simulink model "SF012A_HysCmp"  (R2013b)
settings: Solver=FixedStepDiscrete  StartTime=0.0  StopTime=1  FixedStep=.002  RelTol=1e-3
values from neighbouring files (symbols this model uses):
  ARCHGLBPRM_2MILLISEC_SEC_F32 = DataDict.Constant    [SF012A_HysCmp_DataDict.m]
  EPSILON_ULS_F32 = DataDict.Constant    [SF012A_HysCmp_DataDict.m]
  FLTINJ_HYSCMP_HYSCMPCMD = DataDict.Constant    [SF012A_HysCmp_DataDict.m]
  HysCmpAssiInpLim = DataDict.Calibration    [SF012A_HysCmp_DataDict.m]
  HysCmpOutpLim = DataDict.Calibration    [SF012A_HysCmp_DataDict.m]
  HysCmpRevGain = DataDict.Calibration    [SF012A_HysCmp_DataDict.m]
  HysCmpRiseX = DataDict.Calibration    [SF012A_HysCmp_DataDict.m]
  HysCmpRiseY = DataDict.Calibration    [SF012A_HysCmp_DataDict.m]
  HYSRISEYLIM_ULS_F32 = DataDict.Constant    [SF012A_HysCmp_DataDict.m]
  HYSSATNLOWLIM_HWNWTMTR_F32 = DataDict.Constant    [SF012A_HysCmp_DataDict.m]
  SysGlbPrmSysTqRat = DataDict.ImprtdCal    [SF012A_HysCmp_DataDict.m]
libraries: FixdToFloat x18, FloatToFixd x14, LnrIntrpn x12, NxtrAbslt x10, NxtrLim x8, Fil x6, NxtrSign x5, simulink x2, NxtrMath x1, BilnrIntrpnMplX x1, NxtrMax x1
(part 1 of 2)
settings Model: Creator=TZ5743  LastModifiedBy=TZ5743
settings DataIOCC: LimitDataPoints=off  SaveFormat=Structure  ReturnWorkspaceOutputs=on
settings OptimizationCC: BlockReduction=off  InlineParams=on  ZeroExternalMemoryAtStartup=off  ZeroInternalMemoryAtStartup=off  OptimizeModelRefInitCode=on  LifeSpan=1
settings DebuggingCC: SignalInfNanChecking=error  SignalRangeChecking=warning  UnderspecifiedInitializationDetection=Simplified  SolverPrmCheckMsg=error  InheritedTsInSrcMsg=error  DiscreteInheritContinuousMsg=error  SingleTaskRateTransMsg=error  TasksWithSamePriorityMsg=error  SigSpecEnsureSampleTimeMsg=error  CheckMatrixSingularityMsg=error  IntegerOverflowMsg=error  ParameterUnderflowMsg=error  ParameterPrecisionLossMsg=error  ParameterTunabilityLossMsg=error  FixptConstUnderflowMsg=warning  FixptConstOverflowMsg=warning  VectorMatrixConversionMsg=error  SignalLabelMismatchMsg=error  UnconnectedInputMsg=error  UnconnectedOutputMsg=error  UnconnectedLineMsg=error  SFcnCompatibilityMsg=error  UniqueDataStoreMsg=warning  BusObjectLabelMismatch=error  RootOutportRequireBusObject=error  AssertControl=DisableAll  ModelReferenceIOMsg=error  ModelReferenceVersionMismatchMessage=warning  ModelReferenceIOMismatchMessage=error  ModelReferenceCSMismatchMessage=warning  ModelReferenceDataLoggingMessage=error  StateNameClashWarn=warning  StrictBusMsg=ErrorOnBusTreatedAsVector  NonBusSignalsTreatedAsBus=error  SFUnexpectedBacktrackingDiag=error  SFInvalidInputDataAccessInChartInitDiag=error  SFNoUnconditionalDefaultTransitionDiag=error  SFTransitionOutsideNaturalParentDiag=error  SFUnconditionalTransitionShadowingDiag=error  SFUndirectedBroadcastEventsDiag=error
settings ModelReferenceCC: ModelReferenceNumInstancesAllowed=Single
settings RTWCC: SystemTargetFile=autosar.tlc  GenCodeOnly=on  TemplateMakefile=ert_default_tmf  Description=AUTOSAR  GenerateReport=on  ProcessScript=autosar_make_rtw_hook  LaunchReport=on
settings CodeAppCC: GenerateComments=off  IgnoreCustomStorageClasses=off  CustomSymbolStrType=$N$R$M  CustomSymbolStrBlkIO=$N$M  SimulinkBlockComments=off
settings STFCustomTargetCC: ParMdlRefBuildCompliant=on  CompOptLevelCompliant=on  IncludeMdlTerminateFcn=off  CombineOutputUpdateFcns=on  SuppressErrorStatus=on  ERTFirstTimeCompliant=on  ERTCustomFileBanners=on  SupportNonFinite=off  SupportComplex=off  SupportContinuousTime=off  SupportNonInlinedSFcns=off  MATLABClassNameForMDSCustomization=Simulink.SoftwareTarget.ERTCustomization  AutosarCompliant=on  GRTInterface=off  SystemTargetFile=autosar.tlc
settings ERTTargetCC: CodeReplacementLibrary=ANSI_C  ConcurrentExecutionCompliant=off  IncludeMdlTerminateFcn=off  SuppressErrorStatus=on  SupportNonFinite=off  SupportComplex=off  ModelStepFunctionPrototypeControlCompliant=off  CPPClassGenCompliant=off  AutosarCompliant=on  InlinedParameterPlacement=NonHierarchical  ERTCustomFileTemplate=example_file_process.tlc  EnableUserReplacementTypes=on

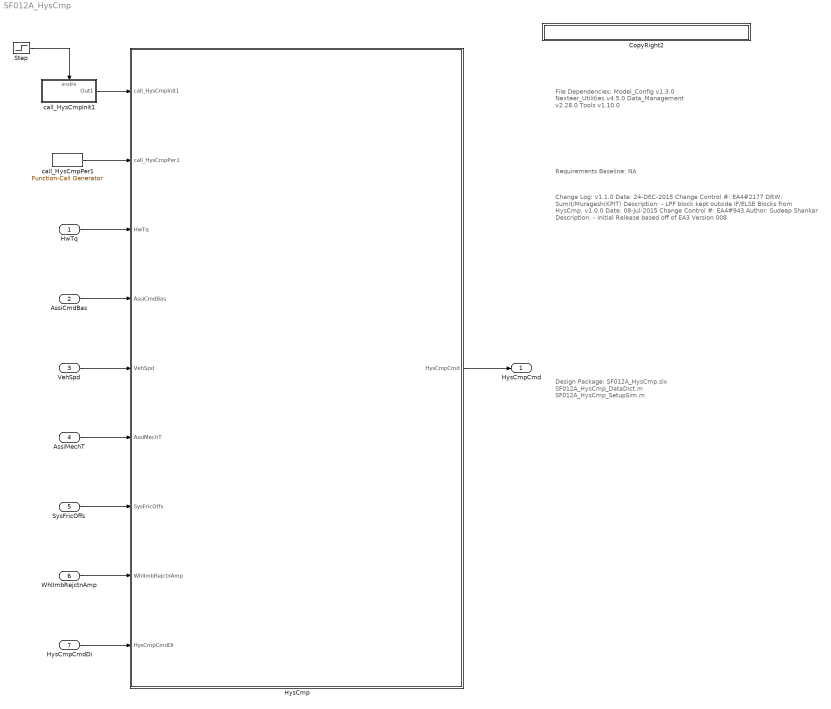
== system SF012A_HysCmp ==
  note: File Dependencies:
      |
      | Model_Config v1.3.0
      | Nexteer_Utilities v4.5.0
      | Data_Management v2.28.0
      | Tools v1.10.0
  note: Requirements Baseline: NA
  note: Change Log:
      | v1.1.0
      | Date: 24-DEC-2015
      | Change Control #: EA4#2177
      | DRW:  Sumit/Muragesh(KPIT)
      | Description:
      | -  LPF block kept outside IF/ELSE Blocks from HysCmp.
      |
      | v1.0.0
      | Date: 08-Jul-2015
      | Change Control #: EA4#943
      | Author:  Sudeep Shankar
      | Description:
      | - Initial Release based off of EA3 Version 008
  note: Design Package:
      |
      | SF012A_HysCmp.slx
      | SF012A_HysCmp_DataDict.m
      | SF012A_HysCmp_SetupSim.m
  HwTq : Inport
  AssiCmdBas : Inport  Port=2
  VehSpd : Inport  Port=3
  AssiMechT : Inport  Port=4
  SysFricOffs : Inport  Port=5
  WhlImbRejctnAmp : Inport  Port=6
  HysCmpCmdDi : Inport  Port=7
  CopyRight2 : Subsystem  Description=|  mask(Copyright Information){none=on}
      | Copyright info block.                                               
      |                                                                     
      | Place copyright information at the top of every subsystem in design.
      mask prompts: none "No parameters"
      mask help: Place copyright information at the top of every subsystem in design.
      mask Display:
      | NxtrConf = 'Nexteer Confidential';
      | 
      | sys = bdroot; %handle for the current model ("system")
      | first = get_param(sys,'Created');
      | if(isempty(first))
      |     first = datestr(now,'yyyy');
      | else
      |     first = first(end-3:end);  %year is last four digits
      | end
      | 
      | last = get_param(sys,'LastModifiedDate');
      | if isempty(last)
      |     last = datestr(now,'yyyy');
      | else
      |     last = last(end-3:end);
      | end
      | 
      | if strcmp(first,last)
      |     fprintf('%s -- Copyright %s Nexteer',NxtrConf,first)
      | else
      |     fprintf('%s -- %s%s- %s Nexteer',NxtrConf,char(169),first,last)
      | end
  HysCmp : Subsystem
  Step : Step  Time=.001  Before=1  After=0  SampleTime=0
  call_HysCmpInit1 : Subsystem  TreatAsAtomicUnit=on
  call_HysCmpPer1 : simulink/Ports & Subsystems/Function-Call Generator  RequirementInfo={} %GIDa_211e4458_5e3d_455a_8408_cf5f2d6f0325  sample_time=0.002  numberOfIterations=1
  HysCmpCmd : Outport
  wires:
  HwTq/1 -> HysCmp/3(HwTq)
  AssiCmdBas/1 -> HysCmp/4(AssiCmdBas)
  VehSpd/1 -> HysCmp/5(VehSpd)
  AssiMechT/1 -> HysCmp/6(AssiMechT)
  SysFricOffs/1 -> HysCmp/7(SysFricOffs)
  WhlImbRejctnAmp/1 -> HysCmp/8(WhlImbRejctnAmp)
  HysCmpCmdDi/1 -> HysCmp/9(HysCmpCmdDi)
  HysCmp/1(HysCmpCmd) -> HysCmpCmd/1
  call_HysCmpPer1/1 -> HysCmp/2(call_HysCmpPer1)
  call_HysCmpInit1/1(Out1) -> HysCmp/1(call_HysCmpInit1)
  Step/1 -> call_HysCmpInit1/Enable

== system SF012A_HysCmp/CopyRight2 ==

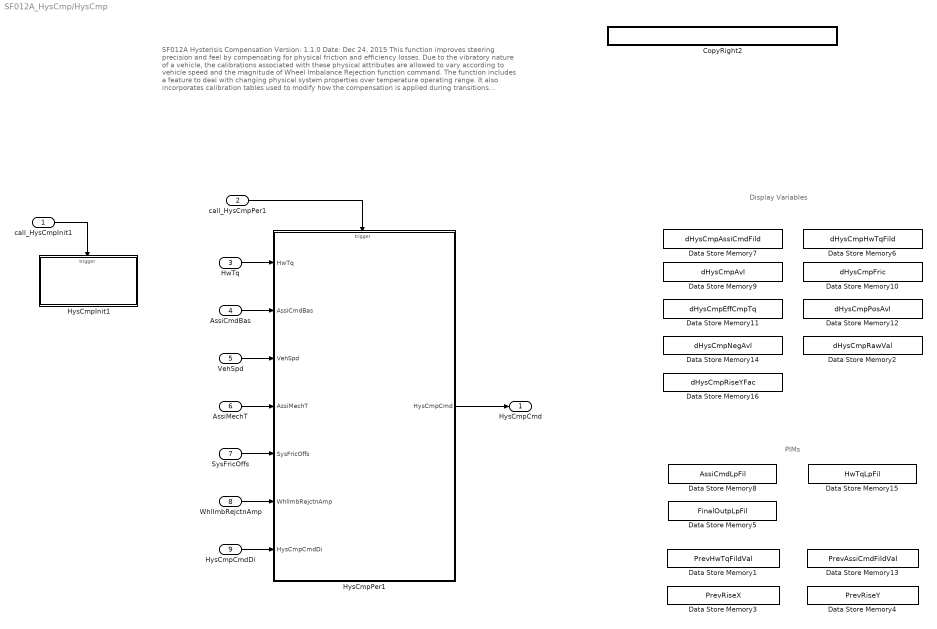
== system SF012A_HysCmp/HysCmp ==
  note: SF012A Hysterisis Compensation       Version: 1.1.0                                                        Date:  Dec 24, 2015
      |
      | This function improves steering precision and feel by compensating for physical friction and efficiency losses.
      | Due to the vibratory nature of a vehicle, the calibrations associated with these physical attributes are allowed
      | to vary according to vehicle speed and the magnitude of Wheel Imbalance Rejection function command. The function
      | includes a feature to deal with changing physical system properties over temperature operating range. It also
      | incorporates calibration tables used to modify how the compensation is applied during transitions between operating
      | quadrants and during periods of near-zero handwheel torque. Finally the function may be disabled for purposes of
      | bench testing
  note: PIMs
  note: Display Variables
  call_HysCmpInit1 : Inport
  call_HysCmpPer1 : Inport  Port=2
  HwTq : Inport  Port=3
  AssiCmdBas : Inport  Port=4
  VehSpd : Inport  Port=5
  AssiMechT : Inport  Port=6
  SysFricOffs : Inport  Port=7
  WhlImbRejctnAmp : Inport  Port=8
  HysCmpCmdDi : Inport  Port=9
  CopyRight2 : Subsystem  Description=|  mask(Copyright Information){none=on}
      | Copyright info block.                                               
      |                                                                     
      | Place copyright information at the top of every subsystem in design.
      mask prompts: none "No parameters"
      mask help: Place copyright information at the top of every subsystem in design.
      mask Display:
      | NxtrConf = 'Nexteer Confidential';
      | 
      | sys = bdroot; %handle for the current model ("system")
      | first = get_param(sys,'Created');
      | if(isempty(first))
      |     first = datestr(now,'yyyy');
      | else
      |     first = first(end-3:end);  %year is last four digits
      | end
      | 
      | last = get_param(sys,'LastModifiedDate');
      | if isempty(last)
      |     last = datestr(now,'yyyy');
      | else
      |     last = last(end-3:end);
      | end
      | 
      | if strcmp(first,last)
      |     fprintf('%s -- Copyright %s Nexteer',NxtrConf,first)
      | else
      |     fprintf('%s -- %s%s- %s Nexteer',NxtrConf,char(169),first,last)
      | end
  Data Store Memory1 : DataStoreMemory  DataStoreName=PrevHwTqFildVal  StateMustResolveToSignalObject=on
  Data Store Memory10 : DataStoreMemory  DataStoreName=dHysCmpFric  ReadBeforeWriteMsg=warning  WriteAfterWriteMsg=warning  WriteAfterReadMsg=warning  StateMustResolveToSignalObject=on
  Data Store Memory11 : DataStoreMemory  DataStoreName=dHysCmpEffCmpTq  ReadBeforeWriteMsg=warning  WriteAfterWriteMsg=warning  WriteAfterReadMsg=warning  StateMustResolveToSignalObject=on
  Data Store Memory12 : DataStoreMemory  DataStoreName=dHysCmpPosAvl  ReadBeforeWriteMsg=warning  WriteAfterWriteMsg=warning  WriteAfterReadMsg=warning  StateMustResolveToSignalObject=on
  Data Store Memory13 : DataStoreMemory  DataStoreName=PrevAssiCmdFildVal  StateMustResolveToSignalObject=on
  Data Store Memory14 : DataStoreMemory  DataStoreName=dHysCmpNegAvl  ReadBeforeWriteMsg=warning  WriteAfterWriteMsg=warning  WriteAfterReadMsg=warning  StateMustResolveToSignalObject=on
  Data Store Memory15 : DataStoreMemory  DataStoreName=HwTqLpFil  InitialValue=struct('FilSt',single(0),'FilGain',single(0))  OutDataTypeStr=Bus: FilLpRec1  StateMustResolveToSignalObject=on
  Data Store Memory16 : DataStoreMemory  DataStoreName=dHysCmpRiseYFac  ReadBeforeWriteMsg=warning  WriteAfterWriteMsg=warning  WriteAfterReadMsg=warning  StateMustResolveToSignalObject=on
  Data Store Memory2 : DataStoreMemory  DataStoreName=dHysCmpRawVal  ReadBeforeWriteMsg=warning  WriteAfterWriteMsg=warning  WriteAfterReadMsg=warning  StateMustResolveToSignalObject=on
  Data Store Memory3 : DataStoreMemory  DataStoreName=PrevRiseX  StateMustResolveToSignalObject=on
  Data Store Memory4 : DataStoreMemory  DataStoreName=PrevRiseY  StateMustResolveToSignalObject=on
  Data Store Memory5 : DataStoreMemory  DataStoreName=FinalOutpLpFil  InitialValue=struct('FilSt',single(0),'FilGain',single(0))  OutDataTypeStr=Bus: FilLpRec1  StateMustResolveToSignalObject=on
  Data Store Memory6 : DataStoreMemory  DataStoreName=dHysCmpHwTqFild  ReadBeforeWriteMsg=warning  WriteAfterWriteMsg=warning  WriteAfterReadMsg=warning  StateMustResolveToSignalObject=on
  Data Store Memory7 : DataStoreMemory  DataStoreName=dHysCmpAssiCmdFild  ReadBeforeWriteMsg=warning  WriteAfterWriteMsg=warning  WriteAfterReadMsg=warning  StateMustResolveToSignalObject=on
  Data Store Memory8 : DataStoreMemory  DataStoreName=AssiCmdLpFil  InitialValue=struct('FilSt',single(0),'FilGain',single(0))  OutDataTypeStr=Bus: FilLpRec1  StateMustResolveToSignalObject=on
  Data Store Memory9 : DataStoreMemory  DataStoreName=dHysCmpAvl  ReadBeforeWriteMsg=warning  WriteAfterWriteMsg=warning  WriteAfterReadMsg=warning  StateMustResolveToSignalObject=on
  HysCmpInit1 : Subsystem
  HysCmpPer1 : Subsystem
  HysCmpCmd : Outport
  wires:
  call_HysCmpInit1/1 -> HysCmpInit1/Trigger
  HwTq/1 -> HysCmpPer1/1(HwTq)
  AssiCmdBas/1 -> HysCmpPer1/2(AssiCmdBas)
  call_HysCmpPer1/1 -> HysCmpPer1/Trigger
  HysCmpPer1/1(HysCmpCmd) -> HysCmpCmd/1
  VehSpd/1 -> HysCmpPer1/3(VehSpd)
  AssiMechT/1 -> HysCmpPer1/4(AssiMechT)
  SysFricOffs/1 -> HysCmpPer1/5(SysFricOffs)
  WhlImbRejctnAmp/1 -> HysCmpPer1/6(WhlImbRejctnAmp)
  HysCmpCmdDi/1 -> HysCmpPer1/7(HysCmpCmdDi)

== system SF012A_HysCmp/call_HysCmpInit1 ==
  Enable : EnablePort
  Function-Call Generator : simulink/Ports & Subsystems/Function-Call Generator  sample_time=.002  numberOfIterations=1
  Out1 : Outport
  wires:
  Function-Call Generator/1 -> Out1/1

== system SF012A_HysCmp/HysCmp/CopyRight2 ==

== system SF012A_HysCmp/HysCmp/HysCmpInit1 ==
  function : TriggerPort  TriggerType=function-call
  CopyRight2 : Subsystem  Description=|  mask(Copyright Information){none=on}
      | Copyright info block.                                               
      |                                                                     
      | Place copyright information at the top of every subsystem in design.
      mask prompts: none "No parameters"
      mask help: Place copyright information at the top of every subsystem in design.
      mask Display:
      | NxtrConf = 'Nexteer Confidential';
      | 
      | sys = bdroot; %handle for the current model ("system")
      | first = get_param(sys,'Created');
      | if(isempty(first))
      |     first = datestr(now,'yyyy');
      | else
      |     first = first(end-3:end);  %year is last four digits
      | end
      | 
      | last = get_param(sys,'LastModifiedDate');
      | if isempty(last)
      |     last = datestr(now,'yyyy');
      | else
      |     last = last(end-3:end);
      | end
      | 
      | if strcmp(first,last)
      |     fprintf('%s -- Copyright %s Nexteer',NxtrConf,first)
      | else
      |     fprintf('%s -- %s%s- %s Nexteer',NxtrConf,char(169),first,last)
      | end
  HysCmpAssiCmdLpFilInit1 : Fil/FilLpInit  Ic=0  Ts=ARCHGLBPRM_2MILLISEC_SEC_F32  Freq=HysCmpAssiCmdLpFilFrq  StVar=AssiCmdLpFil
  HysCmpFinalOutpLpFil1 : Fil/FilLpInit  Ic=0  Ts=ARCHGLBPRM_2MILLISEC_SEC_F32  Freq=HysCmpFinalOutpLpFilFrq  StVar=FinalOutpLpFil
  HysCmpHwTqLpFilInit : Fil/FilLpInit  Ic=0  Ts=ARCHGLBPRM_2MILLISEC_SEC_F32  Freq=HysCmpHwTqLpFilFrq  StVar=HwTqLpFil

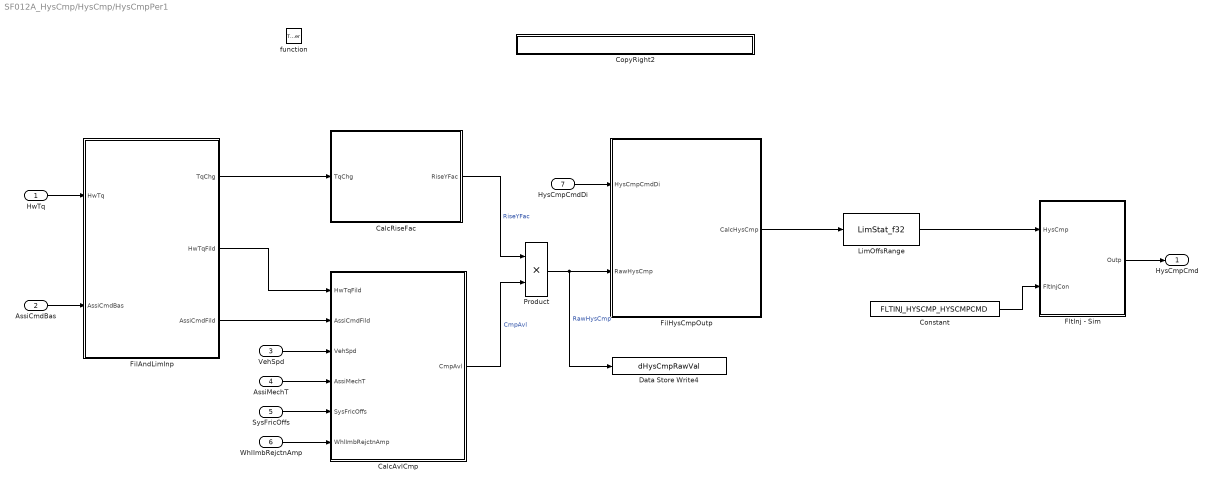
== system SF012A_HysCmp/HysCmp/HysCmpPer1 ==
  HwTq : Inport
  AssiCmdBas : Inport  Port=2
  VehSpd : Inport  Port=3
  AssiMechT : Inport  Port=4
  SysFricOffs : Inport  Port=5
  WhlImbRejctnAmp : Inport  Port=6
  HysCmpCmdDi : Inport  Port=7
  function : TriggerPort  TriggerType=function-call
  CalcAvlCmp : Subsystem
  CalcRiseFac : Subsystem
  Constant : Constant  Value=FLTINJ_HYSCMP_HYSCMPCMD
  CopyRight2 : Subsystem  Description=|  mask(Copyright Information){none=on}
      | Copyright info block.                                               
      |                                                                     
      | Place copyright information at the top of every subsystem in design.
      mask prompts: none "No parameters"
      mask help: Place copyright information at the top of every subsystem in design.
      mask Display:
      | NxtrConf = 'Nexteer Confidential';
      | 
      | sys = bdroot; %handle for the current model ("system")
      | first = get_param(sys,'Created');
      | if(isempty(first))
      |     first = datestr(now,'yyyy');
      | else
      |     first = first(end-3:end);  %year is last four digits
      | end
      | 
      | last = get_param(sys,'LastModifiedDate');
      | if isempty(last)
      |     last = datestr(now,'yyyy');
      | else
      |     last = last(end-3:end);
      | end
      | 
      | if strcmp(first,last)
      |     fprintf('%s -- Copyright %s Nexteer',NxtrConf,first)
      | else
      |     fprintf('%s -- %s%s- %s Nexteer',NxtrConf,char(169),first,last)
      | end
  Data Store Write4 : DataStoreWrite  DataStoreName=dHysCmpRawVal
  FilAndLimInp : Subsystem
  FilHysCmpOutp : Subsystem
  FltInj - Sim : Subsystem  TreatAsAtomicUnit=on  VariantControl=FltInj_sim  mask(Fault_Injection){}
      mask help: Fault Injection is a simulation only block for EA4 programs.
  LimOffsRange : NxtrLim/LimStat_f32  LoLim=SYSGLBPRM_MOTTQCMDLOLIM_MOTNWTMTR_F32  HiLim=SYSGLBPRM_MOTTQCMDHILIM_MOTNWTMTR_F32
      settings: AttributesFormatString=|
      | Low Limit: %<LoLim>
      | High Limit:%<HiLim>
  Product : Product  OutDataTypeStr=Inherit: Inherit via back propagation  RndMeth=Zero
  HysCmpCmd : Outport
  wires:
  HwTq/1 -> FilAndLimInp/1(HwTq)
  AssiCmdBas/1 -> FilAndLimInp/2(AssiCmdBas)
  FilAndLimInp/3(AssiCmdFild) -> CalcAvlCmp/2(AssiCmdFild)
  FilAndLimInp/1(TqChg) -> CalcRiseFac/1(TqChg)
  FilAndLimInp/2(HwTqFild) -> CalcAvlCmp/1(HwTqFild)
  SysFricOffs/1 -> CalcAvlCmp/5(SysFricOffs)
  AssiMechT/1 -> CalcAvlCmp/4(AssiMechT)
  VehSpd/1 -> CalcAvlCmp/3(VehSpd)
  WhlImbRejctnAmp/1 -> CalcAvlCmp/6(WhlImbRejctnAmp)
  CalcRiseFac/1(RiseYFac) -> Product/1  "RiseYFac"
  CalcAvlCmp/1(CmpAvl) -> Product/2  "CmpAvl"
  Product/1 -> FilHysCmpOutp/2(RawHysCmp), Data Store Write4/1  "RawHysCmp"
  HysCmpCmdDi/1 -> FilHysCmpOutp/1(HysCmpCmdDi)
  FilHysCmpOutp/1(CalcHysCmp) -> LimOffsRange/1
  Constant/1 -> FltInj - Sim/2(FltInjCon)
  FltInj - Sim/1(Outp) -> HysCmpCmd/1
  LimOffsRange/1 -> FltInj - Sim/1(HysCmp)

== system SF012A_HysCmp/HysCmp/HysCmpInit1/CopyRight2 ==

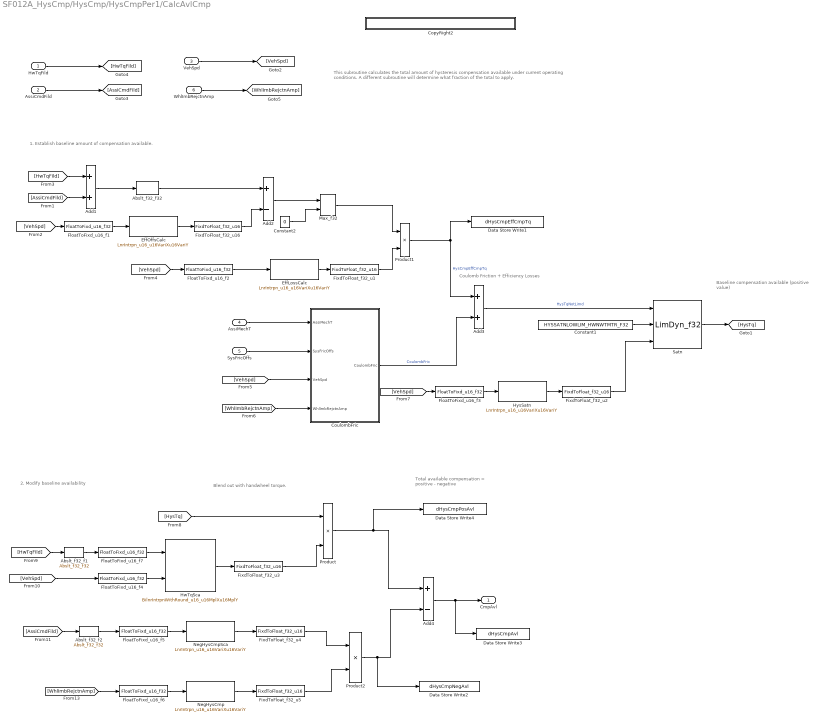
== system SF012A_HysCmp/HysCmp/HysCmpPer1/CalcAvlCmp ==
  note: This subroutine calculates the total amount of hysteresis compensation available under current operating conditions.
      | A different subroutine will determine what fraction of the total to apply.
  note: Total available compensation
      | = positive - negative
  note: Blend out with handwheel torque.
  note: 2. Modify baseline availability
  note: 1. Establish baseline amount of compensation available.
  note: Baseline compensation available
      | (positive value)
  note: Coulomb Friction + Efficiency Losses
  HwTqFild : Inport
  AssiCmdFild : Inport  Port=2
  VehSpd : Inport  Port=3
  AssiMechT : Inport  Port=4
  SysFricOffs : Inport  Port=5
  WhlImbRejctnAmp : Inport  Port=6
  Abslt_f32_f1 : NxtrAbslt/Abslt_f32_f32  SFunctionSpec=single y1 = Abslt_f32_f32(single u1)
      settings: AttributesFormatString=%<Name>
  Abslt_f32_f2 : NxtrAbslt/Abslt_f32_f32  SFunctionSpec=single y1 = Abslt_f32_f32(single u1)
      settings: AttributesFormatString=%<Name>
  Abslt_f32_f32 : NxtrAbslt/Abslt_f32_f32  SFunctionSpec=single y1 = Abslt_f32_f32(single u1)
      settings: AttributesFormatString=%<Name>
  Add1 : Sum  RndMeth=Zero
  Add2 : Sum  Inputs=+-  RndMeth=Zero
  Add3 : Sum  RndMeth=Zero
  Add4 : Sum  Inputs=+-  RndMeth=Zero
  Constant1 : Constant  Value=HYSSATNLOWLIM_HWNWTMTR_F32
  Constant2 : Constant  Value=0  OutDataTypeStr=single
  CopyRight2 : Subsystem  Description=|  mask(Copyright Information){none=on}
      | Copyright info block.                                               
      |                                                                     
      | Place copyright information at the top of every subsystem in design.
      mask prompts: none "No parameters"
      mask help: Place copyright information at the top of every subsystem in design.
      mask Display:
      | NxtrConf = 'Nexteer Confidential';
      | 
      | sys = bdroot; %handle for the current model ("system")
      | first = get_param(sys,'Created');
      | if(isempty(first))
      |     first = datestr(now,'yyyy');
      | else
      |     first = first(end-3:end);  %year is last four digits
      | end
      | 
      | last = get_param(sys,'LastModifiedDate');
      | if isempty(last)
      |     last = datestr(now,'yyyy');
      | else
      |     last = last(end-3:end);
      | end
      | 
      | if strcmp(first,last)
      |     fprintf('%s -- Copyright %s Nexteer',NxtrConf,first)
      | else
      |     fprintf('%s -- %s%s- %s Nexteer',NxtrConf,char(169),first,last)
      | end
  CoulombFric : Subsystem
  Data Store Write1 : DataStoreWrite  DataStoreName=dHysCmpEffCmpTq
  Data Store Write2 : DataStoreWrite  DataStoreName=dHysCmpNegAvl
  Data Store Write3 : DataStoreWrite  DataStoreName=dHysCmpAvl
  Data Store Write4 : DataStoreWrite  DataStoreName=dHysCmpPosAvl
  EffLossCalc : LnrIntrpn/LnrIntrpn_u16_u16VariXu16VariY  XTbl=SysGlbPrmVehSpdBilnrSeln  YTbl=HysCmpEffLossY
      settings: AttributesFormatString=Lnr ( u16VariX , u16VariY )
  EffOffsCalc : LnrIntrpn/LnrIntrpn_u16_u16VariXu16VariY  XTbl=SysGlbPrmVehSpdBilnrSeln  YTbl=HysCmpEffOffsY
      settings: AttributesFormatString=Lnr ( u16VariX , u16VariY )
  FixdToFloat_f32_u1 : FixdToFloat/FixdToFloat_f32_u16  Param1=12
  FixdToFloat_f32_u16 : FixdToFloat/FixdToFloat_f32_u16  Param1=7
  FixdToFloat_f32_u2 : FixdToFloat/FixdToFloat_f32_u16  Param1=7
  FixdToFloat_f32_u3 : FixdToFloat/FixdToFloat_f32_u16  Param1=12
  FixdToFloat_f32_u4 : FixdToFloat/FixdToFloat_f32_u16  Param1=14
  FixdToFloat_f32_u5 : FixdToFloat/FixdToFloat_f32_u16  Param1=7
  FloatToFixd_u16_f{1..5} (5 alike) : FloatToFixd/FloatToFixd_u16_f32  Param1=7
  FloatToFixd_u16_f6 : FloatToFixd/FloatToFixd_u16_f32  Param1=8
  FloatToFixd_u16_f7 : FloatToFixd/FloatToFixd_u16_f32  Param1=12
  HwTqSca : BilnrIntrpnMplX/BilnrIntrpnWithRound_u16_u16MplXu16MplY  MplXTbl=HysCmpHwTqScaX  MplYTbl=HysCmpHwTqScaY  BilnrSelnTbl=SysGlbPrmVehSpdBilnrSeln
      settings: AttributesFormatString=Bilnr ( u16MplX , u16MplY )
  HysSatn : LnrIntrpn/LnrIntrpn_u16_u16VariXu16VariY  XTbl=SysGlbPrmVehSpdBilnrSeln  YTbl=HysCmpHysSatnY
      settings: AttributesFormatString=Lnr ( u16VariX , u16VariY )
  Max_f32 : NxtrMax/Max_f32  SFunctionSpec=single y1 = Max_f32(single u1, single u2)
      settings: AttributesFormatString=%<Name>
  NegHysCmp : LnrIntrpn/LnrIntrpn_u16_u16VariXu16VariY  XTbl=HysCmpNegHysCmpX  YTbl=HysCmpNegHysCmpY
      settings: AttributesFormatString=Lnr ( u16VariX , u16VariY )
  NegHysCmpSca : LnrIntrpn/LnrIntrpn_u16_u16VariXu16VariY  XTbl=HysCmpNegHysCmpScaX  YTbl=HysCmpNegHysCmpScaY
      settings: AttributesFormatString=Lnr ( u16VariX , u16VariY )
  Product : Product  RndMeth=Zero
  Product1 : Product  RndMeth=Zero
  Product2 : Product  RndMeth=Zero
  Satn : NxtrLim/LimDyn_f32
  CmpAvl : Outport
  wires:
  AssiCmdFild/1 -> [AssiCmdFild]
  VehSpd/1 -> [VehSpd]
  HwTqFild/1 -> [HwTqFild]
  WhlImbRejctnAmp/1 -> [WhlImbRejctnAmp]
  [HwTqFild] -> Add1/1
  [AssiCmdFild] -> Add1/2
  Add1/1 -> Abslt_f32_f32/1
  [VehSpd] -> FloatToFixd_u16_f1/1
  Abslt_f32_f32/1 -> Add2/1
  EffOffsCalc/1 -> FixdToFloat_f32_u16/1
  Add2/1 -> Max_f32/1
  Constant2/1 -> Max_f32/2
  [VehSpd] -> FloatToFixd_u16_f2/1
  EffLossCalc/1 -> FixdToFloat_f32_u1/1
  FloatToFixd_u16_f1/1 -> EffOffsCalc/1
  FixdToFloat_f32_u16/1 -> Add2/2
  FloatToFixd_u16_f2/1 -> EffLossCalc/1
  FixdToFloat_f32_u1/1 -> Product1/2
  AssiMechT/1 -> CoulombFric/1(AssiMechT)
  [VehSpd] -> CoulombFric/3(VehSpd)
  SysFricOffs/1 -> CoulombFric/2(SysFricOffs)
  [WhlImbRejctnAmp] -> CoulombFric/4(WhlImbRejctnAmp)
  Product1/1 -> Add3/1, Data Store Write1/1  "HysCmpEffCmpTq"
  CoulombFric/1(CoulombFric) -> Add3/2  "CoulombFric"
  Add3/1 -> Satn/1  "HysTqNotLimd"
  Constant1/1 -> Satn/2
  HysSatn/1 -> FixdToFloat_f32_u2/1
  [VehSpd] -> FloatToFixd_u16_f3/1
  FloatToFixd_u16_f3/1 -> HysSatn/1
  FixdToFloat_f32_u2/1 -> Satn/3
  Satn/1 -> [HysTq]
  [HysTq] -> Product/1
  [HwTqFild] -> Abslt_f32_f1/1
  Abslt_f32_f1/1 -> FloatToFixd_u16_f7/1
  [VehSpd] -> FloatToFixd_u16_f4/1
  HwTqSca/1 -> FixdToFloat_f32_u3/1
  FloatToFixd_u16_f4/1 -> HwTqSca/2
  Product/1 -> Data Store Write4/1, Add4/1
  [AssiCmdFild] -> Abslt_f32_f2/1
  Abslt_f32_f2/1 -> FloatToFixd_u16_f5/1
  FloatToFixd_u16_f5/1 -> NegHysCmpSca/1
  FixdToFloat_f32_u3/1 -> Product/2
  NegHysCmpSca/1 -> FixdToFloat_f32_u4/1
  FixdToFloat_f32_u4/1 -> Product2/1
  [WhlImbRejctnAmp] -> FloatToFixd_u16_f6/1
  FloatToFixd_u16_f6/1 -> NegHysCmp/1
  NegHysCmp/1 -> FixdToFloat_f32_u5/1
  FixdToFloat_f32_u5/1 -> Product2/2
  Product2/1 -> Data Store Write2/1, Add4/2
  Add4/1 -> Data Store Write3/1, CmpAvl/1
  Max_f32/1 -> Product1/1
  FloatToFixd_u16_f7/1 -> HwTqSca/1

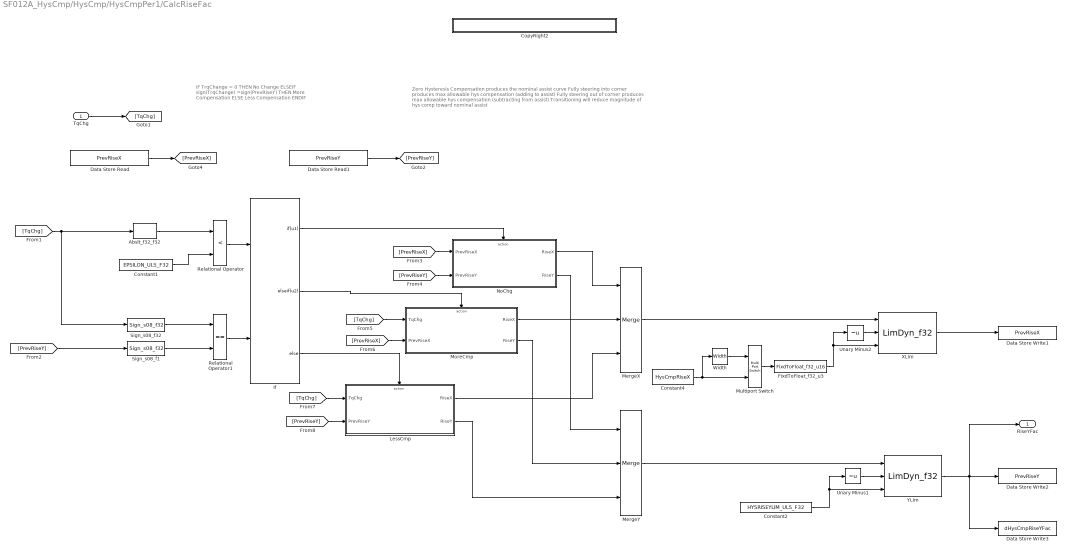
== system SF012A_HysCmp/HysCmp/HysCmpPer1/CalcRiseFac ==
  note: IF TrqChange = 0  THEN
      |      No Change
      | ELSEIF sign(TrqChange) =sign(PrevRiseY)  THEN
      |      More Compensation
      | ELSE
      |      Less Compensation
      | ENDIF
  note: Zero Hysteresis Compensation produces the nominal assist curve
      | Fully steering into corner produces max allowable hys compensation (adding to assist)
      | Fully steering out of corner produces max allowable hys compensation (subtracting from assist)
      | Transitioning will reduce magnitude of hys comp toward nominal assist
  TqChg : Inport
  Abslt_f32_f32 : NxtrAbslt/Abslt_f32_f32  SFunctionSpec=single y1 = Abslt_f32_f32(single u1)
      settings: AttributesFormatString=%<Name>
  Constant1 : Constant  Value=EPSILON_ULS_F32
  Constant2 : Constant  Value=HYSRISEYLIM_ULS_F32
  Constant4 : Constant  Value=HysCmpRiseX
  CopyRight2 : Subsystem  Description=|  mask(Copyright Information){none=on}
      | Copyright info block.                                               
      |                                                                     
      | Place copyright information at the top of every subsystem in design.
      mask prompts: none "No parameters"
      mask help: Place copyright information at the top of every subsystem in design.
      mask Display:
      | NxtrConf = 'Nexteer Confidential';
      | 
      | sys = bdroot; %handle for the current model ("system")
      | first = get_param(sys,'Created');
      | if(isempty(first))
      |     first = datestr(now,'yyyy');
      | else
      |     first = first(end-3:end);  %year is last four digits
      | end
      | 
      | last = get_param(sys,'LastModifiedDate');
      | if isempty(last)
      |     last = datestr(now,'yyyy');
      | else
      |     last = last(end-3:end);
      | end
      | 
      | if strcmp(first,last)
      |     fprintf('%s -- Copyright %s Nexteer',NxtrConf,first)
      | else
      |     fprintf('%s -- %s%s- %s Nexteer',NxtrConf,char(169),first,last)
      | end
  Data Store Read : DataStoreRead  DataStoreName=PrevRiseX
  Data Store Read1 : DataStoreRead  DataStoreName=PrevRiseY
  Data Store Write1 : DataStoreWrite  DataStoreName=PrevRiseX
  Data Store Write2 : DataStoreWrite  DataStoreName=PrevRiseY
  Data Store Write3 : DataStoreWrite  DataStoreName=dHysCmpRiseYFac
  FixdToFloat_f32_u3 : FixdToFloat/FixdToFloat_f32_u16  Param1=14
  If : If  NumInputs=2  IfExpression=u1  ElseIfExpressions=u2
  LessCmp : Subsystem  TreatAsAtomicUnit=on
  MergeX : Merge  Inputs=3
  MergeY : Merge  Inputs=3
  MoreCmp : Subsystem  TreatAsAtomicUnit=on
  Multiport Switch : MultiPortSwitch  Inputs=1
  NoChg : Subsystem  TreatAsAtomicUnit=on
  Relational Operator : RelationalOperator  Operator=<  OutDataTypeStr=boolean
  Relational Operator1 : RelationalOperator  Operator===  OutDataTypeStr=boolean
  Sign_s08_f1 : NxtrSign/Sign_s08_f32  SFunctionSpec=int8 y1 = Sign_s08_f32(single u1)
  Sign_s08_f32 : NxtrSign/Sign_s08_f32  SFunctionSpec=int8 y1 = Sign_s08_f32(single u1)
  Unary Minus1 : UnaryMinus
  Unary Minus2 : UnaryMinus
  Width : Width  DataType=uint16
  XLim : NxtrLim/LimDyn_f32
  YLim : NxtrLim/LimDyn_f32
  RiseYFac : Outport
  wires:
  Sign_s08_f1/1 -> Relational Operator1/2
  If/2 -> MoreCmp/Action
  If/3 -> LessCmp/Action
  [TqChg] -> Sign_s08_f32/1, Abslt_f32_f32/1
  Sign_s08_f32/1 -> Relational Operator1/1
  If/1 -> NoChg/Action
  TqChg/1 -> [TqChg]
  NoChg/1(RiseX) -> MergeX/1
  MoreCmp/1(RiseX) -> MergeX/2
  LessCmp/1(RiseX) -> MergeX/3
  NoChg/2(RiseY) -> MergeY/1
  MoreCmp/2(RiseY) -> MergeY/2
  LessCmp/2(RiseY) -> MergeY/3
  MergeX/1 -> XLim/1
  MergeY/1 -> YLim/1
  FixdToFloat_f32_u3/1 -> XLim/3, Unary Minus2/1
  Unary Minus2/1 -> XLim/2
  Unary Minus1/1 -> YLim/2
  Data Store Read/1 -> [PrevRiseX]
  Data Store Read1/1 -> [PrevRiseY]
  [PrevRiseY] -> Sign_s08_f1/1
  [PrevRiseX] -> NoChg/1(PrevRiseX)
  [PrevRiseY] -> NoChg/2(PrevRiseY)
  [TqChg] -> MoreCmp/1(TqChg)
  [PrevRiseX] -> MoreCmp/2(PrevRiseX)
  [TqChg] -> LessCmp/1(TqChg)
  [PrevRiseY] -> LessCmp/2(PrevRiseY)
  Constant4/1 -> Multiport Switch/2, Width/1
  Width/1 -> Multiport Switch/1
  Multiport Switch/1 -> FixdToFloat_f32_u3/1
  YLim/1 -> Data Store Write3/1, Data Store Write2/1, RiseYFac/1
  XLim/1 -> Data Store Write1/1
  Constant2/1 -> YLim/3, Unary Minus1/1
  Relational Operator/1 -> If/1
  Abslt_f32_f32/1 -> Relational Operator/1
  Constant1/1 -> Relational Operator/2
  Relational Operator1/1 -> If/2

== system SF012A_HysCmp/HysCmp/HysCmpPer1/CopyRight2 ==

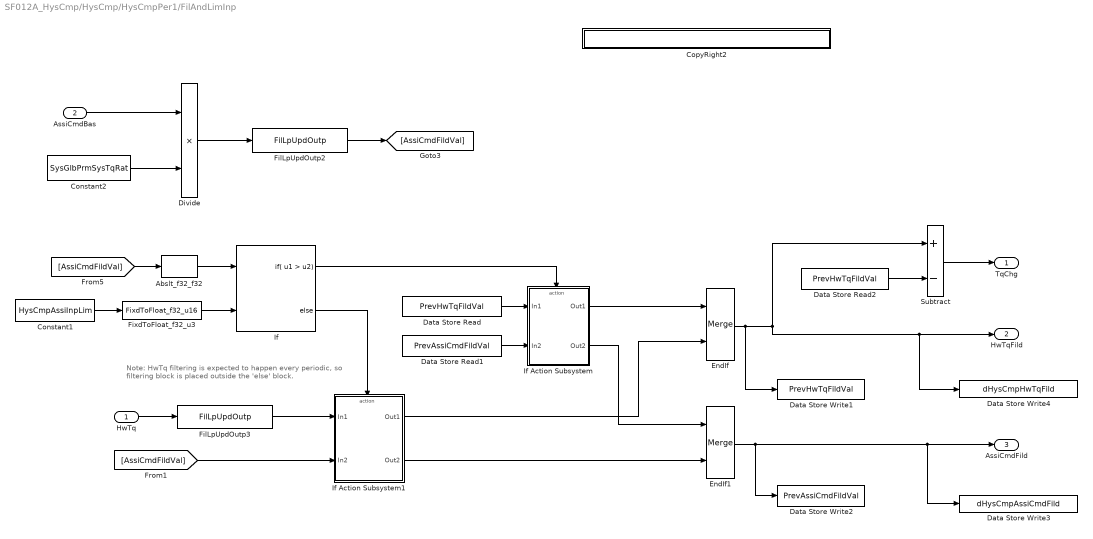
== system SF012A_HysCmp/HysCmp/HysCmpPer1/FilAndLimInp ==
  note: Note:
      | HwTq filtering is expected to happen every periodic, so filtering
      | block is placed outside the 'else' block.
  HwTq : Inport
  AssiCmdBas : Inport  Port=2
  Abslt_f32_f32 : NxtrAbslt/Abslt_f32_f32  SFunctionSpec=single y1 = Abslt_f32_f32(single u1)
      settings: AttributesFormatString=%<Name>
  Constant1 : Constant  Value=HysCmpAssiInpLim
  Constant2 : Constant  Value=SysGlbPrmSysTqRat
  CopyRight2 : Subsystem  Description=|  mask(Copyright Information){none=on}
      | Copyright info block.                                               
      |                                                                     
      | Place copyright information at the top of every subsystem in design.
      mask prompts: none "No parameters"
      mask help: Place copyright information at the top of every subsystem in design.
      mask Display:
      | NxtrConf = 'Nexteer Confidential';
      | 
      | sys = bdroot; %handle for the current model ("system")
      | first = get_param(sys,'Created');
      | if(isempty(first))
      |     first = datestr(now,'yyyy');
      | else
      |     first = first(end-3:end);  %year is last four digits
      | end
      | 
      | last = get_param(sys,'LastModifiedDate');
      | if isempty(last)
      |     last = datestr(now,'yyyy');
      | else
      |     last = last(end-3:end);
      | end
      | 
      | if strcmp(first,last)
      |     fprintf('%s -- Copyright %s Nexteer',NxtrConf,first)
      | else
      |     fprintf('%s -- %s%s- %s Nexteer',NxtrConf,char(169),first,last)
      | end
  Data Store Read : DataStoreRead  DataStoreName=PrevHwTqFildVal
  Data Store Read1 : DataStoreRead  DataStoreName=PrevAssiCmdFildVal
  Data Store Read2 : DataStoreRead  DataStoreName=PrevHwTqFildVal
  Data Store Write1 : DataStoreWrite  DataStoreName=PrevHwTqFildVal
  Data Store Write2 : DataStoreWrite  DataStoreName=PrevAssiCmdFildVal
  Data Store Write3 : DataStoreWrite  DataStoreName=dHysCmpAssiCmdFild
  Data Store Write4 : DataStoreWrite  DataStoreName=dHysCmpHwTqFild
  Divide : Product
  EndIf : Merge
  EndIf1 : Merge
  FilLpUpdOutp2 : Fil/FilLpUpdOutp  StVar=AssiCmdLpFil
      settings: AttributesFormatString=StVar: %<StVar>
  FilLpUpdOutp3 : Fil/FilLpUpdOutp  StVar=HwTqLpFil
      settings: AttributesFormatString=StVar: %<StVar>
  FixdToFloat_f32_u3 : FixdToFloat/FixdToFloat_f32_u16  Param1=7
  If : If  NumInputs=2  IfExpression=u1 > u2
  If Action Subsystem : Subsystem  TreatAsAtomicUnit=on
  If Action Subsystem1 : Subsystem  TreatAsAtomicUnit=on
  Subtract : Sum  Inputs=+-  RndMeth=Zero
  TqChg : Outport
  HwTqFild : Outport  Port=2
  AssiCmdFild : Outport  Port=3
  wires:
  FilLpUpdOutp2/1 -> [AssiCmdFildVal]
  Divide/1 -> FilLpUpdOutp2/1
  AssiCmdBas/1 -> Divide/1
  Constant2/1 -> Divide/2
  [AssiCmdFildVal] -> Abslt_f32_f32/1
  Abslt_f32_f32/1 -> If/1
  Constant1/1 -> FixdToFloat_f32_u3/1
  If/1 -> If Action Subsystem/Action
  If/2 -> If Action Subsystem1/Action
  HwTq/1 -> FilLpUpdOutp3/1
  [AssiCmdFildVal] -> If Action Subsystem1/2(In2)
  FilLpUpdOutp3/1 -> If Action Subsystem1/1(In1)
  If Action Subsystem1/1(Out1) -> EndIf/2
  If Action Subsystem/1(Out1) -> EndIf/1
  Data Store Read/1 -> If Action Subsystem/1(In1)
  Data Store Read1/1 -> If Action Subsystem/2(In2)
  If Action Subsystem/2(Out2) -> EndIf1/1
  If Action Subsystem1/2(Out2) -> EndIf1/2
  Subtract/1 -> TqChg/1
  EndIf/1 -> Data Store Write1/1, Data Store Write4/1, HwTqFild/1, Subtract/1
  Data Store Read2/1 -> Subtract/2
  EndIf1/1 -> Data Store Write3/1, AssiCmdFild/1, Data Store Write2/1
  FixdToFloat_f32_u3/1 -> If/2

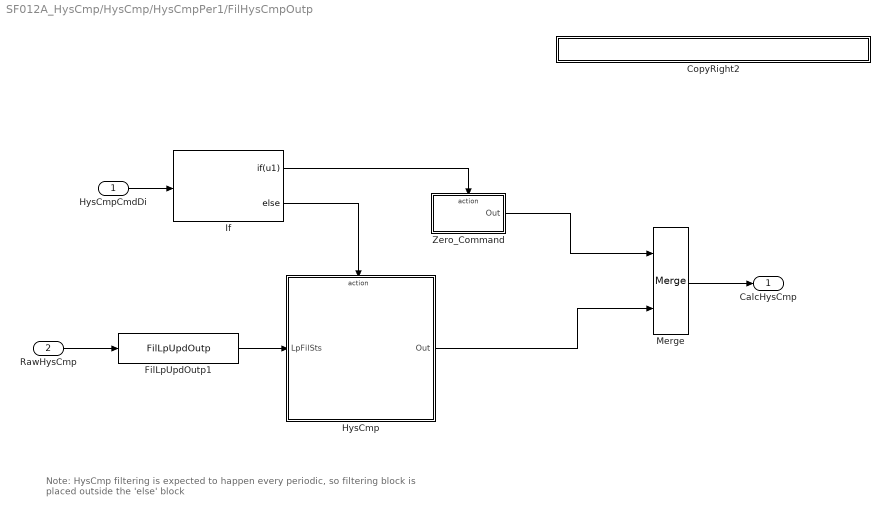
== system SF012A_HysCmp/HysCmp/HysCmpPer1/FilHysCmpOutp ==
  note: Note:
      | HysCmp filtering is expected to happen every periodic, so filtering block is placed
      | outside the 'else' block
  HysCmpCmdDi : Inport
  RawHysCmp : Inport  Port=2
  CopyRight2 : Subsystem  Description=|  mask(Copyright Information){none=on}
      | Copyright info block.                                               
      |                                                                     
      | Place copyright information at the top of every subsystem in design.
      mask prompts: none "No parameters"
      mask help: Place copyright information at the top of every subsystem in design.
      mask Display:
      | NxtrConf = 'Nexteer Confidential';
      | 
      | sys = bdroot; %handle for the current model ("system")
      | first = get_param(sys,'Created');
      | if(isempty(first))
      |     first = datestr(now,'yyyy');
      | else
      |     first = first(end-3:end);  %year is last four digits
      | end
      | 
      | last = get_param(sys,'LastModifiedDate');
      | if isempty(last)
      |     last = datestr(now,'yyyy');
      | else
      |     last = last(end-3:end);
      | end
      | 
      | if strcmp(first,last)
      |     fprintf('%s -- Copyright %s Nexteer',NxtrConf,first)
      | else
      |     fprintf('%s -- %s%s- %s Nexteer',NxtrConf,char(169),first,last)
      | end
  FilLpUpdOutp1 : Fil/FilLpUpdOutp  StVar=FinalOutpLpFil
      settings: AttributesFormatString=StVar: %<StVar>
  HysCmp : Subsystem  RequirementInfo={} %GIDa_95224ba3_d373_47aa_9e2d_c8f1beaf79f1  TreatAsAtomicUnit=on
  If : If  RequirementInfo={} %GIDa_94a310f4_6e32_4cd6_8e0d_2a7931f46409  IfExpression=u1
  Merge : Merge
  Zero_Command : Subsystem  RequirementInfo={} %GIDa_7dfea39b_76f9_4579_a42d_48172b08e8b5  TreatAsAtomicUnit=on
  CalcHysCmp : Outport
  wires:
  HysCmp/1(Out) -> Merge/2
  If/1 -> Zero_Command/Action
  If/2 -> HysCmp/Action
  HysCmpCmdDi/1 -> If/1
  Zero_Command/1(Out) -> Merge/1
  Merge/1 -> CalcHysCmp/1
  RawHysCmp/1 -> FilLpUpdOutp1/1
  FilLpUpdOutp1/1 -> HysCmp/1(LpFilSts)

== system SF012A_HysCmp/HysCmp/HysCmpPer1/FltInj - Sim ==
  note: Inport #2 must be Constant
  note: EA4.x Fault Injection
  note: This block requires no modification by FDD author.
      |
      | This block does not actually simulate any fault injection.  It is simply a pass-thru.
      |
      | The port (#2) simply terminates its signal, but we are trying to force the FDD author
      | to properly use the Constant in FDD model.
  HysCmp : Inport
  FltInjCon : Inport  Port=2
  CopyRight2 : Subsystem  Description=|  mask(Copyright Information){none=on}
      | Copyright info block.                                               
      |                                                                     
      | Place copyright information at the top of every subsystem in design.
      mask prompts: none "No parameters"
      mask help: Place copyright information at the top of every subsystem in design.
      mask Display:
      | NxtrConf = 'Nexteer Confidential';
      | 
      | sys = bdroot; %handle for the current model ("system")
      | first = get_param(sys,'Created');
      | if(isempty(first))
      |     first = datestr(now,'yyyy');
      | else
      |     first = first(end-3:end);  %year is last four digits
      | end
      | 
      | last = get_param(sys,'LastModifiedDate');
      | if isempty(last)
      |     last = datestr(now,'yyyy');
      | else
      |     last = last(end-3:end);
      | end
      | 
      | if strcmp(first,last)
      |     fprintf('%s -- Copyright %s Nexteer',NxtrConf,first)
      | else
      |     fprintf('%s -- %s%s- %s Nexteer',NxtrConf,char(169),first,last)
      | end
  Terminator : Terminator
  Outp : Outport
  wires:
  FltInjCon/1 -> Terminator/1
  HysCmp/1 -> Outp/1

== system SF012A_HysCmp/HysCmp/HysCmpPer1/CalcAvlCmp/CopyRight2 ==

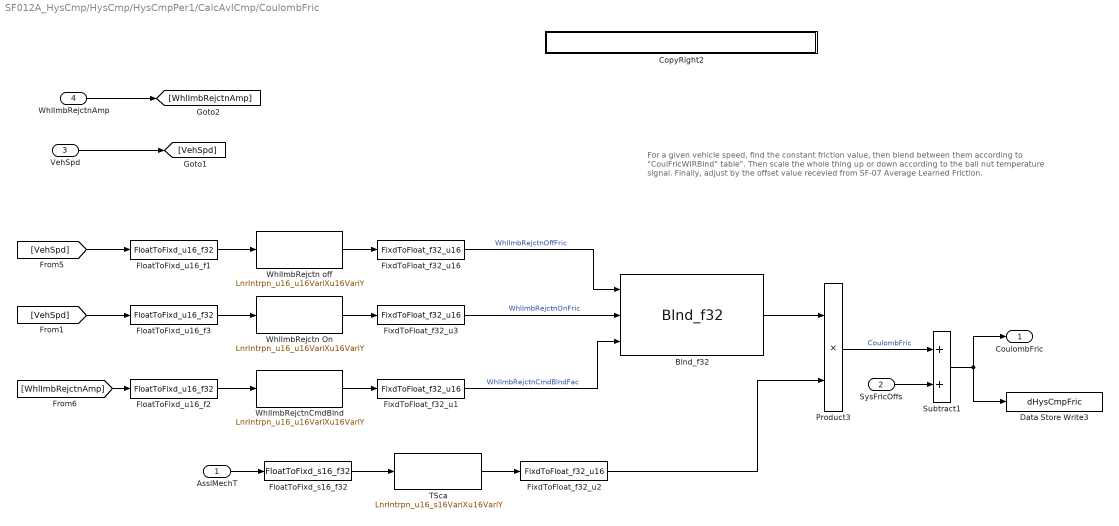
== system SF012A_HysCmp/HysCmp/HysCmpPer1/CalcAvlCmp/CoulombFric ==
  note: For a given vehicle speed, find the constant friction value, then blend between them
      | according to "CoulFricWIRBlnd" table".
      |
      | Then scale the whole thing up or down according to the ball nut temperature signal.
      |
      | Finally, adjust by the offset value recevied from SF-07 Average Learned Friction.
  AssiMechT : Inport
  SysFricOffs : Inport  Port=2
  VehSpd : Inport  Port=3
  WhlImbRejctnAmp : Inport  Port=4
  Blnd_f32 : NxtrMath/Blnd_f32  SFunctionSpec=single y1 = Blnd_f32(single u1, single u2, single u3)  Parameter3=on
      settings: AttributesFormatString=%<Name>
  CopyRight2 : Subsystem  Description=|  mask(Copyright Information){none=on}
      | Copyright info block.                                               
      |                                                                     
      | Place copyright information at the top of every subsystem in design.
      mask prompts: none "No parameters"
      mask help: Place copyright information at the top of every subsystem in design.
      mask Display:
      | NxtrConf = 'Nexteer Confidential';
      | 
      | sys = bdroot; %handle for the current model ("system")
      | first = get_param(sys,'Created');
      | if(isempty(first))
      |     first = datestr(now,'yyyy');
      | else
      |     first = first(end-3:end);  %year is last four digits
      | end
      | 
      | last = get_param(sys,'LastModifiedDate');
      | if isempty(last)
      |     last = datestr(now,'yyyy');
      | else
      |     last = last(end-3:end);
      | end
      | 
      | if strcmp(first,last)
      |     fprintf('%s -- Copyright %s Nexteer',NxtrConf,first)
      | else
      |     fprintf('%s -- %s%s- %s Nexteer',NxtrConf,char(169),first,last)
      | end
  Data Store Write3 : DataStoreWrite  DataStoreName=dHysCmpFric
  FixdToFloat_f32_u1 : FixdToFloat/FixdToFloat_f32_u16  Param1=14
  FixdToFloat_f32_u16 : FixdToFloat/FixdToFloat_f32_u16  Param1=7
  FixdToFloat_f32_u2 : FixdToFloat/FixdToFloat_f32_u16  Param1=7
  FixdToFloat_f32_u3 : FixdToFloat/FixdToFloat_f32_u16  Param1=7
  FloatToFixd_s16_f32 : FloatToFixd/FloatToFixd_s16_f32  Param1=1
  FloatToFixd_u16_f1 : FloatToFixd/FloatToFixd_u16_f32  Param1=7
  FloatToFixd_u16_f2 : FloatToFixd/FloatToFixd_u16_f32  Param1=8
  FloatToFixd_u16_f3 : FloatToFixd/FloatToFixd_u16_f32  Param1=7
  Product3 : Product  RndMeth=Zero
  Subtract1 : Sum
  TSca : LnrIntrpn/LnrIntrpn_u16_s16VariXu16VariY  XTbl=HysCmpFricTScaX  YTbl=HysCmpFricTScaY
      settings: AttributesFormatString=Lnr ( s16VariX , u16VariY )
  WhlImbRejctn On : LnrIntrpn/LnrIntrpn_u16_u16VariXu16VariY  XTbl=SysGlbPrmVehSpdBilnrSeln  YTbl=HysCmpFricWhlImbRejctnOnY
      settings: AttributesFormatString=Lnr ( u16VariX , u16VariY )
  WhlImbRejctn off : LnrIntrpn/LnrIntrpn_u16_u16VariXu16VariY  XTbl=SysGlbPrmVehSpdBilnrSeln  YTbl=HysCmpFricWhlImbRejctnOffY
      settings: AttributesFormatString=Lnr ( u16VariX , u16VariY )
  WhlImbRejctnCmdBlnd : LnrIntrpn/LnrIntrpn_u16_u16VariXu16VariY  XTbl=HysCmpFricWhlImbRejctnBlndX  YTbl=HysCmpFricWhlImbRejctnBlndY
      settings: AttributesFormatString=Lnr ( u16VariX , u16VariY )
  CoulombFric : Outport
  wires:
  AssiMechT/1 -> FloatToFixd_s16_f32/1
  SysFricOffs/1 -> Subtract1/2
  VehSpd/1 -> [VehSpd]
  WhlImbRejctnAmp/1 -> [WhlImbRejctnAmp]
  FloatToFixd_s16_f32/1 -> TSca/1
  TSca/1 -> FixdToFloat_f32_u2/1
  FixdToFloat_f32_u2/1 -> Product3/2
  Product3/1 -> Subtract1/1  "CoulombFric"
  Subtract1/1 -> Data Store Write3/1, CoulombFric/1
  [VehSpd] -> FloatToFixd_u16_f1/1
  FloatToFixd_u16_f1/1 -> WhlImbRejctn off/1
  WhlImbRejctnCmdBlnd/1 -> FixdToFloat_f32_u1/1
  [WhlImbRejctnAmp] -> FloatToFixd_u16_f2/1
  FixdToFloat_f32_u16/1 -> Blnd_f32/1  "WhlImbRejctnOffFric"
  FloatToFixd_u16_f2/1 -> WhlImbRejctnCmdBlnd/1
  FixdToFloat_f32_u1/1 -> Blnd_f32/3  "WhlImbRejctnCmdBlndFac"
  [VehSpd] -> FloatToFixd_u16_f3/1
  FloatToFixd_u16_f3/1 -> WhlImbRejctn On/1
  FixdToFloat_f32_u3/1 -> Blnd_f32/2  "WhlImbRejctnOnFric"
  WhlImbRejctn On/1 -> FixdToFloat_f32_u3/1
  WhlImbRejctn off/1 -> FixdToFloat_f32_u16/1
  Blnd_f32/1 -> Product3/1

== system SF012A_HysCmp/HysCmp/HysCmpPer1/CalcRiseFac/CopyRight2 ==

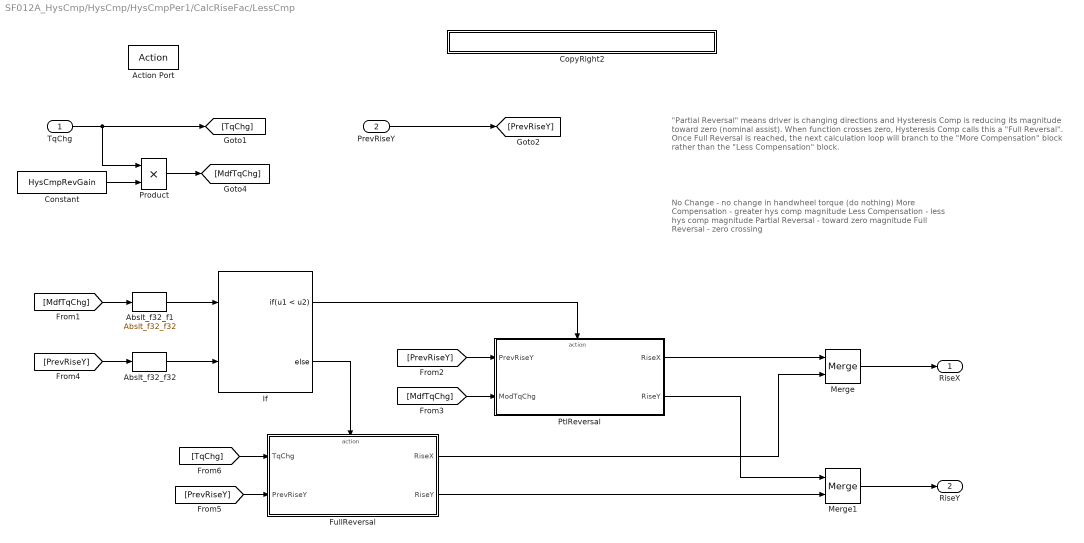
== system SF012A_HysCmp/HysCmp/HysCmpPer1/CalcRiseFac/LessCmp ==
  note: No Change                    - no change in handwheel torque (do nothing)
      |
      | More Compensation     - greater hys comp magnitude
      |
      | Less Compensation     - less hys comp magnitude
      |        Partial Reversal          - toward zero magnitude
      |        Full Reversal               - zero crossing
  note: "Partial Reversal" means driver is changing directions and Hysteresis Comp is reducing its magnitude toward
      | zero (nominal assist).  When function crosses zero, Hysteresis Comp calls this a "Full Reversal".  Once
      | Full Reversal is reached, the next calculation loop will branch to the "More Compensation" block rather
      | than the "Less Compensation" block.
  TqChg : Inport
  PrevRiseY : Inport  Port=2
  Action Port : ActionPort  ActionType=else
  Abslt_f32_f1 : NxtrAbslt/Abslt_f32_f32  SFunctionSpec=single y1 = Abslt_f32_f32(single u1)
      settings: AttributesFormatString=%<Name>
  Abslt_f32_f32 : NxtrAbslt/Abslt_f32_f32  SFunctionSpec=single y1 = Abslt_f32_f32(single u1)
      settings: AttributesFormatString=%<Name>
  Constant : Constant  Value=HysCmpRevGain
  CopyRight2 : Subsystem  Description=|  mask(Copyright Information){none=on}
      | Copyright info block.                                               
      |                                                                     
      | Place copyright information at the top of every subsystem in design.
      mask prompts: none "No parameters"
      mask help: Place copyright information at the top of every subsystem in design.
      mask Display:
      | NxtrConf = 'Nexteer Confidential';
      | 
      | sys = bdroot; %handle for the current model ("system")
      | first = get_param(sys,'Created');
      | if(isempty(first))
      |     first = datestr(now,'yyyy');
      | else
      |     first = first(end-3:end);  %year is last four digits
      | end
      | 
      | last = get_param(sys,'LastModifiedDate');
      | if isempty(last)
      |     last = datestr(now,'yyyy');
      | else
      |     last = last(end-3:end);
      | end
      | 
      | if strcmp(first,last)
      |     fprintf('%s -- Copyright %s Nexteer',NxtrConf,first)
      | else
      |     fprintf('%s -- %s%s- %s Nexteer',NxtrConf,char(169),first,last)
      | end
  FullReversal : Subsystem  TreatAsAtomicUnit=on
  If : If  NumInputs=2  IfExpression=u1 < u2
  Merge : Merge
  Merge1 : Merge
  Product : Product  RndMeth=Zero
  PtlReversal : Subsystem  TreatAsAtomicUnit=on
  RiseX : Outport
  RiseY : Outport  Port=2
  wires:
  TqChg/1 -> Product/1, [TqChg]
  PrevRiseY/1 -> [PrevRiseY]
  Product/1 -> [MdfTqChg]
  [PrevRiseY] -> Abslt_f32_f32/1
  Abslt_f32_f32/1 -> If/2
  [MdfTqChg] -> Abslt_f32_f1/1
  Abslt_f32_f1/1 -> If/1
  If/1 -> PtlReversal/Action
  If/2 -> FullReversal/Action
  [PrevRiseY] -> PtlReversal/1(PrevRiseY)
  [MdfTqChg] -> PtlReversal/2(ModTqChg)
  [PrevRiseY] -> FullReversal/2(PrevRiseY)
  [TqChg] -> FullReversal/1(TqChg)
  PtlReversal/1(RiseX) -> Merge/1
  PtlReversal/2(RiseY) -> Merge1/1
  Merge/1 -> RiseX/1
  Merge1/1 -> RiseY/1
  FullReversal/1(RiseX) -> Merge/2
  FullReversal/2(RiseY) -> Merge1/2
  Constant/1 -> Product/2

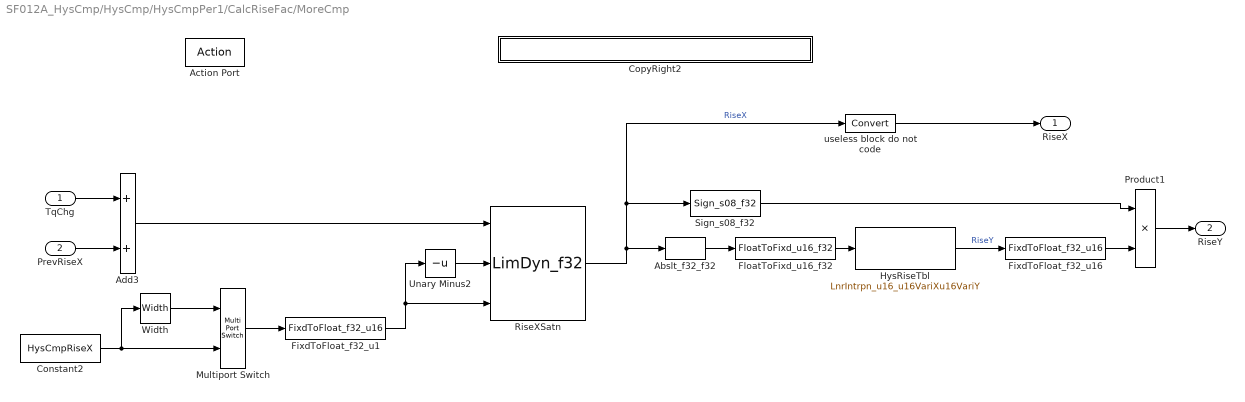
== system SF012A_HysCmp/HysCmp/HysCmpPer1/CalcRiseFac/MoreCmp ==
  TqChg : Inport
  PrevRiseX : Inport  Port=2
  Action Port : ActionPort  ActionType=elseif
  Abslt_f32_f32 : NxtrAbslt/Abslt_f32_f32  SFunctionSpec=single y1 = Abslt_f32_f32(single u1)
      settings: AttributesFormatString=%<Name>
  Add3 : Sum  RndMeth=Zero
  Constant2 : Constant  Value=HysCmpRiseX
  CopyRight2 : Subsystem  Description=|  mask(Copyright Information){none=on}
      | Copyright info block.                                               
      |                                                                     
      | Place copyright information at the top of every subsystem in design.
      mask prompts: none "No parameters"
      mask help: Place copyright information at the top of every subsystem in design.
      mask Display:
      | NxtrConf = 'Nexteer Confidential';
      | 
      | sys = bdroot; %handle for the current model ("system")
      | first = get_param(sys,'Created');
      | if(isempty(first))
      |     first = datestr(now,'yyyy');
      | else
      |     first = first(end-3:end);  %year is last four digits
      | end
      | 
      | last = get_param(sys,'LastModifiedDate');
      | if isempty(last)
      |     last = datestr(now,'yyyy');
      | else
      |     last = last(end-3:end);
      | end
      | 
      | if strcmp(first,last)
      |     fprintf('%s -- Copyright %s Nexteer',NxtrConf,first)
      | else
      |     fprintf('%s -- %s%s- %s Nexteer',NxtrConf,char(169),first,last)
      | end
  FixdToFloat_f32_u1 : FixdToFloat/FixdToFloat_f32_u16  Param1=14
  FixdToFloat_f32_u16 : FixdToFloat/FixdToFloat_f32_u16  Param1=14
  FloatToFixd_u16_f32 : FloatToFixd/FloatToFixd_u16_f32  Param1=14
  HysRiseTbl : LnrIntrpn/LnrIntrpn_u16_u16VariXu16VariY  XTbl=HysCmpRiseX  YTbl=HysCmpRiseY
      settings: AttributesFormatString=Lnr ( u16VariX , u16VariY )
  Multiport Switch : MultiPortSwitch  Inputs=1
  Product1 : Product  RndMeth=Zero
  RiseXSatn : NxtrLim/LimDyn_f32
  Sign_s08_f32 : NxtrSign/Sign_s08_f32  SFunctionSpec=int8 y1 = Sign_s08_f32(single u1)
  Unary Minus2 : UnaryMinus
  Width : Width  DataType=uint16
  useless block do not code : DataTypeConversion
  RiseX : Outport
  RiseY : Outport  Port=2
  wires:
  PrevRiseX/1 -> Add3/2
  TqChg/1 -> Add3/1
  Add3/1 -> RiseXSatn/1
  Constant2/1 -> Multiport Switch/2, Width/1
  Unary Minus2/1 -> RiseXSatn/2
  RiseXSatn/1 -> Sign_s08_f32/1, useless block do not code/1, Abslt_f32_f32/1  "RiseX"
  Sign_s08_f32/1 -> Product1/1
  Abslt_f32_f32/1 -> FloatToFixd_u16_f32/1
  HysRiseTbl/1 -> FixdToFloat_f32_u16/1  "RiseY"
  Product1/1 -> RiseY/1
  FloatToFixd_u16_f32/1 -> HysRiseTbl/1
  FixdToFloat_f32_u16/1 -> Product1/2
  Width/1 -> Multiport Switch/1
  Multiport Switch/1 -> FixdToFloat_f32_u1/1
  FixdToFloat_f32_u1/1 -> Unary Minus2/1, RiseXSatn/3
  useless block do not code/1 -> RiseX/1

== system SF012A_HysCmp/HysCmp/HysCmpPer1/CalcRiseFac/NoChg ==
  PrevRiseX : Inport
  PrevRiseY : Inport  Port=2
  Action Port : ActionPort  ActionType=then
  CopyRight2 : Subsystem  Description=|  mask(Copyright Information){none=on}
      | Copyright info block.                                               
      |                                                                     
      | Place copyright information at the top of every subsystem in design.
      mask prompts: none "No parameters"
      mask help: Place copyright information at the top of every subsystem in design.
      mask Display:
      | NxtrConf = 'Nexteer Confidential';
      | 
      | sys = bdroot; %handle for the current model ("system")
      | first = get_param(sys,'Created');
      | if(isempty(first))
      |     first = datestr(now,'yyyy');
      | else
      |     first = first(end-3:end);  %year is last four digits
      | end
      | 
      | last = get_param(sys,'LastModifiedDate');
      | if isempty(last)
      |     last = datestr(now,'yyyy');
      | else
      |     last = last(end-3:end);
      | end
      | 
      | if strcmp(first,last)
      |     fprintf('%s -- Copyright %s Nexteer',NxtrConf,first)
      | else
      |     fprintf('%s -- %s%s- %s Nexteer',NxtrConf,char(169),first,last)
      | end
  RiseX : Outport
  RiseY : Outport  Port=2
  wires:
  PrevRiseX/1 -> RiseX/1
  PrevRiseY/1 -> RiseY/1

== system SF012A_HysCmp/HysCmp/HysCmpPer1/FilAndLimInp/CopyRight2 ==

== system SF012A_HysCmp/HysCmp/HysCmpPer1/FilAndLimInp/If Action Subsystem ==
  In1 : Inport
  In2 : Inport  Port=2
  Action Port : ActionPort  ActionType=then
  CopyRight2 : Subsystem  Description=|  mask(Copyright Information){none=on}
      | Copyright info block.                                               
      |                                                                     
      | Place copyright information at the top of every subsystem in design.
      mask prompts: none "No parameters"
      mask help: Place copyright information at the top of every subsystem in design.
      mask Display:
      | NxtrConf = 'Nexteer Confidential';
      | 
      | sys = bdroot; %handle for the current model ("system")
      | first = get_param(sys,'Created');
      | if(isempty(first))
      |     first = datestr(now,'yyyy');
      | else
      |     first = first(end-3:end);  %year is last four digits
      | end
      | 
      | last = get_param(sys,'LastModifiedDate');
      | if isempty(last)
      |     last = datestr(now,'yyyy');
      | else
      |     last = last(end-3:end);
      | end
      | 
      | if strcmp(first,last)
      |     fprintf('%s -- Copyright %s Nexteer',NxtrConf,first)
      | else
      |     fprintf('%s -- %s%s- %s Nexteer',NxtrConf,char(169),first,last)
      | end
  Out1 : Outport
  Out2 : Outport  Port=2
  wires:
  In1/1 -> Out1/1
  In2/1 -> Out2/1

== system SF012A_HysCmp/HysCmp/HysCmpPer1/FilAndLimInp/If Action Subsystem1 ==
  In1 : Inport
  In2 : Inport  Port=2
  Action Port : ActionPort  ActionType=else
  CopyRight2 : Subsystem  Description=|  mask(Copyright Information){none=on}
      | Copyright info block.                                               
      |                                                                     
      | Place copyright information at the top of every subsystem in design.
      mask prompts: none "No parameters"
      mask help: Place copyright information at the top of every subsystem in design.
      mask Display:
      | NxtrConf = 'Nexteer Confidential';
      | 
      | sys = bdroot; %handle for the current model ("system")
      | first = get_param(sys,'Created');
      | if(isempty(first))
      |     first = datestr(now,'yyyy');
      | else
      |     first = first(end-3:end);  %year is last four digits
      | end
      | 
      | last = get_param(sys,'LastModifiedDate');
      | if isempty(last)
      |     last = datestr(now,'yyyy');
      | else
      |     last = last(end-3:end);
      | end
      | 
      | if strcmp(first,last)
      |     fprintf('%s -- Copyright %s Nexteer',NxtrConf,first)
      | else
      |     fprintf('%s -- %s%s- %s Nexteer',NxtrConf,char(169),first,last)
      | end
  Out1 : Outport
  Out2 : Outport  Port=2
  wires:
  In1/1 -> Out1/1
  In2/1 -> Out2/1
